simulink model "SignalToNoise"  (Simulink 6.5)
settings: Solver=FixedStepDiscrete  StartTime=0.0  StopTime=5  RelTol=1e-3
PreLoadFcn:
  | load dspwlets;
PostLoadFcn:
  | c6000demoscallback
undefined symbols (not defined in the file or in its folder): D, fdesignblkfcn, gcbh
libraries: dspsigops x33, dspstat3 x5, dspsrcs4 x2, dspmathops x2, dspbuff3 x1, dspsigattribs x1
CloseFcn:
  | clear fs hid hir lod lor noisdopp ts;
settings Model: RequirementInfo=9  Creator=don  LastModifiedBy=Administrator  CovMetricSettings=d  ExtModeTrigMode=oneshot  ExtModeArmWhenConnect=off  ProdHWDeviceType=TI C6000
settings SolverCC: PositivePriorityOrder=on
settings DataIOCC: LimitDataPoints=off  SaveOutput=off  SaveTime=off  SignalLoggingName=sigsOut
settings OptimizationCC: BlockReduction=off  BooleanDataType=off  InlineParams=on  InlineInvariantSignals=on  RollThreshold=2  OptimizeModelRefInitCode=on  LifeSpan=1  BufferReusableBoundary=off
settings DebuggingCC: CheckExecutionContextPreStartOutputMsg=on  CheckExecutionContextRuntimeOutputMsg=on  SolverPrmCheckMsg=none  InheritedTsInSrcMsg=none  MultiTaskDSMMsg=warning  MultiTaskCondExecSysMsg=none  IntegerOverflowMsg=none  StrictBusMsg=None
settings HardwareCC: ProdBitPerLong=40  ProdIntDivRoundTo=Zero  ProdEndianess=LittleEndian  ProdHWDeviceType=TI C6000  TargetHWDeviceType=32-bit Generic
settings ModelReferenceCC: UpdateModelReferenceTargets=IfOutOfDate
settings RTWCC: SystemTargetFile=ti_c6000_ert.tlc  GenCodeOnly=on  TemplateMakefile=ti_c6000_ert.tmf  ProcessScript=ti_c6000_ert_make_rtw_hook  IncludeERTFirstTime=on
settings CodeAppCC: IgnoreCustomStorageClasses=off  PrefixModelToSubsysFcnNames=off  CustomSymbolStrFcn=$F$N$M
settings C6000ERTTargetCC: TargetFcnLib=ansi_tfl_tmw.mat  GenFloatMathFcnCalls=ANSI_C  UtilityFuncGeneration=Auto  GenerateFullHeader=on  GenerateSampleERTMain=on  GenerateTestInterfaces=off  IsPILTarget=off  ModelReferenceCompliant=off  IncludeMdlTerminateFcn=on  CombineOutputUpdateFcns=on  SuppressErrorStatus=off  IncludeFileDelimiter=Auto  ERTCustomFileBanners=on  SupportAbsoluteTime=on  LogVarNameModifier=rt_  MatFileLogging=off  MultiInstanceERTCode=off  SupportNonFinite=on  SupportComplex=on  PurelyIntegerCode=off  SupportContinuousTime=on  SupportNonInlinedSFcns=on  EnableShiftOperators=on  ParenthesesLevel=Nominal  GenerateErtSFunction=off  GenerateASAP2=off  ExtMode=off  ExtModeTransport=0  ExtModeStaticAlloc=off  ExtModeStaticAllocSize=1000000  ExtModeTesting=off  ExtModeMexFile=ext_comm  InlinedParameterPlacement=NonHierarchical  TargetOS=BareBoardExample  MultiInstanceErrorCode=Error  RateGroupingCode=on  RootIOFormat=Individual arguments  RTWCAPISignals=off  RTWCAPIParams=off  RTWCAPIStates=off  ERTSrcFileBannerTemplate=ert_code_template.cgt  ERTHdrFileBannerTemplate=ert_code_template.cgt  ERTDataSrcFileTemplate=ert_code_template.cgt  ERTDataHdrFileTemplate=ert_code_template.cgt  ERTCustomFileTemplate=example_file_process.tlc  ModuleNamingRule=Unspecified  SignalDisplayLevel=10  ParamTuneLevel=10  GlobalDataDefinition=Auto  DataDefinitionFile=global.c  GlobalDataReference=Auto  DataReferenceFile=global.h  GRTInterface=off  EnableUserReplacementTypes=off  MemSecPackage=--- None ---  MemSecDataConstants=Default  MemSecDataIO=Default  MemSecDataInternal=Default  MemSecDataParameters=Default  MemSecFuncInitTerm=Default  MemSecFuncExecute=Default  exportCCSObj=on  ccsObjName=CCS_Obj  useDSPBIOS=on  ProfileGenCode=off  InlineDSPBlks=on  FPopt=off  memModel=Far_Aggregate  optLevel=Function(-o2)  CompilerVerbosity=Quiet  InterruptThreshOnC6x=off  SymbolicDebugOnC6x=off  RetainAsmFiles=off  RetainObjFiles=on  CreateMapFile=on  UserStackSize=8192  c6000BuildAction=Build_and_execute  OverrunAction=Notify_and_continue  OverrunNotificationMethod=Turn_on_LEDs

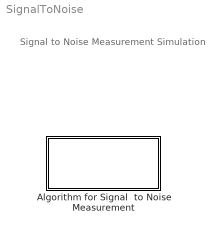
== system SignalToNoise ==
  note: Signal to Noise Measurement Simulation
  Algorithm for Signal  to Noise Measurement : Subsystem  TreatAsAtomicUnit=on

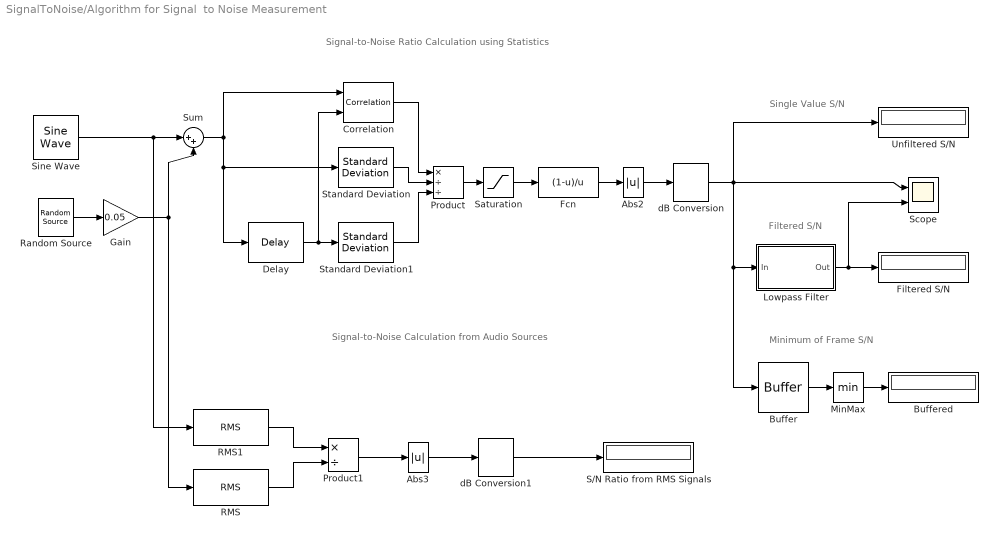
== system SignalToNoise/Algorithm for Signal  to Noise Measurement ==
  note: Signal-to-Noise Ratio Calculation using Statistics
  note: Signal-to-Noise Calculation from Audio Sources
  note: Single Value S/N
  note: Filtered S/N
  note: Minimum of Frame S/N
  Abs2 : Abs  SampleTime=-1  SaturateOnIntegerOverflow=off
  Abs3 : Abs  SampleTime=-1  SaturateOnIntegerOverflow=off
  Buffer : dspbuff3/Buffer  N=16  V=0  ic=0
  "Buffered " : Display
  Correlation : dspstat3/Correlation  DialogController=dspDDGCreate  DialogControllerArgs=DataTag0  domain=Time  roundingMode=Floor  overflowMode=off
  Delay : dspsigops/Delay  dly_unit=Samples  delay=22  ic_detail=off  dif_ic_for_ch=off  dif_ic_for_dly=off  ic=0  reset_popup=None
  Fcn : Fcn  Expr=(1-u)/u
  Filtered S/N : Display
  Gain : Gain  Gain=0.05
  Lowpass Filter : Subsystem  DialogController=fdesignblkfcn  DialogControllerArgs=DataTag2  InitFcn=fdesignblkfcn(gcbh, {'InitFcn'});
      settings: CopyFcn=fdesignblkfcn(gcbh, {'CopyFcn'});
      mask Type: Lowpass Filter
      mask Description: Design a lowpass filter
      mask Help: helpview(mapfilelocation('dspblks'), 'dsplowpassfilter')
      mask Display: disp('Lowpass')
  MinMax : MinMax
  Product : Product  Inputs=*//  RndMeth=Zero
  Product1 : Product  Inputs=*/  RndMeth=Zero
  RMS : dspstat3/RMS  run=on  reset_popup=None
  RMS1 : dspstat3/RMS  run=on  reset_popup=None
  Random Source : dspsrcs4/Random Source  SrcType=Uniform  NormMethod=Ziggurat  CltLength=12  MinVal=0  MaxVal=1  MeanVal=0  VarVal=1  RepMode=Not repeatable  rawSeed=1  IsInherit=off  SampMode=Discrete  SampTime=1/8000  SampFrame=128  DataType=Single  OutComplex=Real
  S/N Ratio from RMS Signals : Display
  Saturation : Saturate  UpperLimit=0.99  LowerLimit=-0.99
  Scope : Scope  NumInputPorts=2
      settings: TimeRange=5  YMin=0~0  YMax=50~30
  Sine Wave : dspsrcs4/Sine Wave  Amplitude=1  Frequency=500  Phase=0  SampleMode=Discrete  OutComplex=Real  CompMethod=Trigonometric fcn  TableSize=Speed  SampleTime=1/8000  SamplesPerFrame=128  dataType=single  wordLen=16  udDataType=sfix(16)  fracBitsMode=Best precision  numFracBits=15  ResetState=Restart at time zero
  Standard Deviation : dspstat3/Standard Deviation  run=off  reset_popup=None
  Standard Deviation1 : dspstat3/Standard Deviation  run=off  reset_popup=None
  Sum : Sum  Inputs=|++
  Unfiltered S/N : Display
  dB Conversion : dspmathops/dB Conversion  SystemSampleTime=-1  dBtype=dB  intype=Power  R=1  fuzz=off
  dB Conversion1 : dspmathops/dB Conversion  SystemSampleTime=-1  dBtype=dB  intype=Power  R=1  fuzz=off
  wires:
  Delay/1 -> Standard Deviation1/1, Correlation/2
  Standard Deviation1/1 -> Product/3
  Random Source/1 -> Gain/1
  Sine Wave/1 -> Sum/1, RMS1/1
  Gain/1 -> Sum/2, RMS/1
  Product/1 -> Saturation/1
  Saturation/1 -> Fcn/1
  Fcn/1 -> Abs2/1
  Abs2/1 -> dB Conversion/1
  Standard Deviation/1 -> Product/2
  Correlation/1 -> Product/1
  Sum/1 -> Correlation/1, Delay/1, Standard Deviation/1
  Product1/1 -> Abs3/1
  dB Conversion/1 -> Scope/1, Unfiltered S/N/1, Buffer/1, Lowpass Filter/1(In)
  dB Conversion1/1 -> S/N Ratio from RMS Signals/1
  RMS/1 -> Product1/2
  RMS1/1 -> Product1/1
  Abs3/1 -> dB Conversion1/1
  Buffer/1 -> MinMax/1
  MinMax/1 -> "Buffered "/1
  Lowpass Filter/1(Out) -> Scope/2, Filtered S/N/1

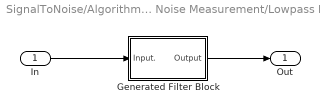
== system SignalToNoise/Algorithm for Signal  to Noise Measurement/Lowpass Filter ==
  In : Inport
  Generated Filter Block : Subsystem  Tag=FilterWizardSubSystem
      settings: ErrorFcn=dspFilterRealizedInBasicElemsAlgLoopErrFcnCallback
  Out : Outport
  wires:
  In/1 -> Generated Filter Block/1(Input.)
  Generated Filter Block/1(Output) -> Out/1

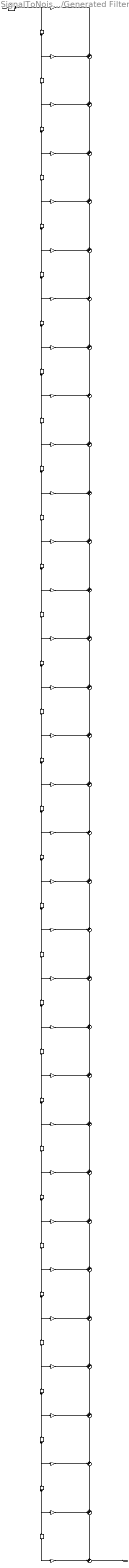
== system SignalToNoise/Algorithm for Signal  to Noise Measurement/Lowpass Filter/Generated Filter Block ==
  Input. : Inport
  BodyDelay{2..33} (32 alike) : dspsigops/Delay  Orientation=down  dly_unit=Samples  delay=1  ic_detail=off  dif_ic_for_ch=off  dif_ic_for_dly=off  ic=0  reset_popup=None
  BodyLSum{2..32} (31 alike) : Sum  Orientation=down  Inputs=++|  RndMeth=Nearest  SaturateOnIntegerOverflow=on  InputSameDT=on
  BodyLSum33 : Sum  Inputs=++|  RndMeth=Nearest  SaturateOnIntegerOverflow=on  InputSameDT=on
  Input : dspsigattribs/Check Signal Attributes  SystemSampleTime=-1  SigAttribCheckMethod=Matches attributes exactly  Complexity=Ignore  Frame=Ignore  DimsCheckMethod=Ignore  Dimensions=1-D  DatatypeCheckMethod=Is not...  DatatypeGeneral=Floating-point  DtypeFloatSpecific=Any floating-point  DtypeFixedSpecific=Any fixed-point  DtypeIntSpecific=Any integer  SampleMode=Ignore
  b(1) : Gain  Gain=0.0031354400327103979  SaturateOnIntegerOverflow=on
  b(10) : Gain  Gain=0.035789149589047442  SaturateOnIntegerOverflow=on
  b(11) : Gain  Gain=0.041576706855248266  SaturateOnIntegerOverflow=on
  b(12) : Gain  Gain=0.047034795573112312  SaturateOnIntegerOverflow=on
  b(13) : Gain  Gain=0.051910996806067158  SaturateOnIntegerOverflow=on
  b(14) : Gain  Gain=0.055974012215601346  SaturateOnIntegerOverflow=on
  b(15) : Gain  Gain=0.059027528615569473  SaturateOnIntegerOverflow=on
  b(16) : Gain  Gain=0.060922094777746717  SaturateOnIntegerOverflow=on
  b(17) : Gain  Gain=0.061564221078339532  SaturateOnIntegerOverflow=on
  b(18) : Gain  Gain=0.060922094777746717  SaturateOnIntegerOverflow=on
  b(19) : Gain  Gain=0.059027528615569473  SaturateOnIntegerOverflow=on
  b(2) : Gain  Gain=0.0036960980168448806  SaturateOnIntegerOverflow=on
  b(20) : Gain  Gain=0.055974012215601346  SaturateOnIntegerOverflow=on
  b(21) : Gain  Gain=0.051910996806067158  SaturateOnIntegerOverflow=on
  b(22) : Gain  Gain=0.047034795573112312  SaturateOnIntegerOverflow=on
  b(23) : Gain  Gain=0.041576706855248266  SaturateOnIntegerOverflow=on
  b(24) : Gain  Gain=0.035789149589047442  SaturateOnIntegerOverflow=on
  b(25) : Gain  Gain=0.029930727273299446  SaturateOnIntegerOverflow=on
  b(26) : Gain  Gain=0.024251199589990391  SaturateOnIntegerOverflow=on
  b(27) : Gain  Gain=0.018977335698013843  SaturateOnIntegerOverflow=on
  b(28) : Gain  Gain=0.0143005509937024  SaturateOnIntegerOverflow=on
  b(29) : Gain  Gain=0.010367095514306547  SaturateOnIntegerOverflow=on
  b(3) : Gain  Gain=0.0050527806983788797  SaturateOnIntegerOverflow=on
  b(30) : Gain  Gain=0.0072713772111905658  SaturateOnIntegerOverflow=on
  b(31) : Gain  Gain=0.0050527806983788797  SaturateOnIntegerOverflow=on
  b(32) : Gain  Gain=0.0036960980168448806  SaturateOnIntegerOverflow=on
  b(33) : Gain  Gain=0.0031354400327103979  SaturateOnIntegerOverflow=on
  b(4) : Gain  Gain=0.0072713772111905658  SaturateOnIntegerOverflow=on
  b(5) : Gain  Gain=0.010367095514306547  SaturateOnIntegerOverflow=on
  b(6) : Gain  Gain=0.0143005509937024  SaturateOnIntegerOverflow=on
  b(7) : Gain  Gain=0.018977335698013843  SaturateOnIntegerOverflow=on
  b(8) : Gain  Gain=0.024251199589990391  SaturateOnIntegerOverflow=on
  b(9) : Gain  Gain=0.029930727273299446  SaturateOnIntegerOverflow=on
  Output : Outport
  wires:
  Input./1 -> Input/1
  Input/1 -> b(1)/1, BodyDelay2/1
  b(1)/1 -> BodyLSum2/2
  BodyDelay2/1 -> b(2)/1, BodyDelay3/1
  b(2)/1 -> BodyLSum2/1
  BodyLSum2/1 -> BodyLSum3/2
  BodyDelay3/1 -> b(3)/1, BodyDelay4/1
  b(3)/1 -> BodyLSum3/1
  BodyLSum3/1 -> BodyLSum4/2
  BodyDelay4/1 -> b(4)/1, BodyDelay5/1
  b(4)/1 -> BodyLSum4/1
  BodyLSum4/1 -> BodyLSum5/2
  BodyDelay5/1 -> b(5)/1, BodyDelay6/1
  b(5)/1 -> BodyLSum5/1
  BodyLSum5/1 -> BodyLSum6/2
  BodyDelay6/1 -> b(6)/1, BodyDelay7/1
  b(6)/1 -> BodyLSum6/1
  BodyLSum6/1 -> BodyLSum7/2
  BodyDelay7/1 -> b(7)/1, BodyDelay8/1
  b(7)/1 -> BodyLSum7/1
  BodyLSum7/1 -> BodyLSum8/2
  BodyDelay8/1 -> b(8)/1, BodyDelay9/1
  b(8)/1 -> BodyLSum8/1
  BodyLSum8/1 -> BodyLSum9/2
  BodyDelay9/1 -> b(9)/1, BodyDelay10/1
  b(9)/1 -> BodyLSum9/1
  BodyLSum9/1 -> BodyLSum10/2
  BodyDelay10/1 -> b(10)/1, BodyDelay11/1
  b(10)/1 -> BodyLSum10/1
  BodyLSum10/1 -> BodyLSum11/2
  BodyDelay11/1 -> b(11)/1, BodyDelay12/1
  b(11)/1 -> BodyLSum11/1
  BodyLSum11/1 -> BodyLSum12/2
  BodyDelay12/1 -> b(12)/1, BodyDelay13/1
  b(12)/1 -> BodyLSum12/1
  BodyLSum12/1 -> BodyLSum13/2
  BodyDelay13/1 -> b(13)/1, BodyDelay14/1
  b(13)/1 -> BodyLSum13/1
  BodyLSum13/1 -> BodyLSum14/2
  BodyDelay14/1 -> b(14)/1, BodyDelay15/1
  b(14)/1 -> BodyLSum14/1
  BodyLSum14/1 -> BodyLSum15/2
  BodyDelay15/1 -> b(15)/1, BodyDelay16/1
  b(15)/1 -> BodyLSum15/1
  BodyLSum15/1 -> BodyLSum16/2
  BodyDelay16/1 -> b(16)/1, BodyDelay17/1
  b(16)/1 -> BodyLSum16/1
  BodyLSum16/1 -> BodyLSum17/2
  BodyDelay17/1 -> b(17)/1, BodyDelay18/1
  b(17)/1 -> BodyLSum17/1
  BodyLSum17/1 -> BodyLSum18/2
  BodyDelay18/1 -> b(18)/1, BodyDelay19/1
  b(18)/1 -> BodyLSum18/1
  BodyLSum18/1 -> BodyLSum19/2
  BodyDelay19/1 -> b(19)/1, BodyDelay20/1
  b(19)/1 -> BodyLSum19/1
  BodyLSum19/1 -> BodyLSum20/2
  BodyDelay20/1 -> b(20)/1, BodyDelay21/1
  b(20)/1 -> BodyLSum20/1
  BodyLSum20/1 -> BodyLSum21/2
  BodyDelay21/1 -> b(21)/1, BodyDelay22/1
  b(21)/1 -> BodyLSum21/1
  BodyLSum21/1 -> BodyLSum22/2
  BodyDelay22/1 -> b(22)/1, BodyDelay23/1
  b(22)/1 -> BodyLSum22/1
  BodyLSum22/1 -> BodyLSum23/2
  BodyDelay23/1 -> b(23)/1, BodyDelay24/1
  b(23)/1 -> BodyLSum23/1
  BodyLSum23/1 -> BodyLSum24/2
  BodyDelay24/1 -> b(24)/1, BodyDelay25/1
  b(24)/1 -> BodyLSum24/1
  BodyLSum24/1 -> BodyLSum25/2
  BodyDelay25/1 -> b(25)/1, BodyDelay26/1
  b(25)/1 -> BodyLSum25/1
  BodyLSum25/1 -> BodyLSum26/2
  BodyDelay26/1 -> b(26)/1, BodyDelay27/1
  b(26)/1 -> BodyLSum26/1
  BodyLSum26/1 -> BodyLSum27/2
  BodyDelay27/1 -> b(27)/1, BodyDelay28/1
  b(27)/1 -> BodyLSum27/1
  BodyLSum27/1 -> BodyLSum28/2
  BodyDelay28/1 -> b(28)/1, BodyDelay29/1
  b(28)/1 -> BodyLSum28/1
  BodyLSum28/1 -> BodyLSum29/2
  BodyDelay29/1 -> b(29)/1, BodyDelay30/1
  b(29)/1 -> BodyLSum29/1
  BodyLSum29/1 -> BodyLSum30/2
  BodyDelay30/1 -> b(30)/1, BodyDelay31/1
  b(30)/1 -> BodyLSum30/1
  BodyLSum30/1 -> BodyLSum31/2
  BodyDelay31/1 -> b(31)/1, BodyDelay32/1
  b(31)/1 -> BodyLSum31/1
  BodyLSum31/1 -> BodyLSum32/2
  BodyDelay32/1 -> b(32)/1, BodyDelay33/1
  b(32)/1 -> BodyLSum32/1
  BodyLSum32/1 -> BodyLSum33/1
  BodyDelay33/1 -> b(33)/1
  b(33)/1 -> BodyLSum33/2
  BodyLSum33/1 -> Output/1
